simulink model "model4_cm"  (R2018b)
settings: Solver=FixedStepDiscrete  StartTime=0.0  StopTime=Inf  FixedStep=0.025  RelTol=1e-3  EnableMultiTasking=on
undefined symbols (not defined in the file): acA2000, Ace, Basler, FreeRun, ipaddr, PoCL, PTP, USETHISONE
libraries: ptplib x5, dotFinder_ul x2, xpcbitflowlib x1, slrtlib x1, xpcutilitieslib x1, xpcrtudplib x1, videoStream_ul x1, imageUDPNode_ul x1
settings Model: sg_rtwmakecfg_data=_bitflow_  SimulationMode=external  Creator=mcobb  LastModifiedBy=MAE-NCSUCORE
settings SolverCC: ConcurrentTasks=on  AutoInsertRateTranBlk=on
settings DataIOCC: SaveFormat=StructureWithTime
settings OptimizationCC: BlockReduction=off  OptimizeBlockIOStorage=off  BufferReuse=off  GlobalBufferReuse=off  ExpressionFolding=off  LocalBlockOutputs=off  OptimizeDataStoreBuffers=off  BusAssignmentInplaceUpdate=off
settings DebuggingCC: LibraryContextMissingDiagnostic=none
settings HardwareCC: ProdBitPerPointer=32  ProdBitPerSizeT=32  ProdBitPerPtrDiffT=32  ProdLargestAtomicFloat=None  ProdWordSize=32  ProdLongLongMode=on  ProdHWDeviceType=Generic->32-bit x86 compatible
settings SFSimCC: SimUseLocalCustomCode=off
settings RTWCC: SystemTargetFile=slrt.tlc  TemplateMakefile=slrt_default_tmf  Description=Simulink Real-Time  RTWUseLocalCustomCode=off  CodeExecutionProfiling=on  RTWCompilerOptimization=on
settings SimulinkRealTimeCC: SupportVariableSizeSignals=on  PreserveStateflowLocalDataDimensions=off  RL32LogTETModifier=off  xPCisDefaultEnv=off  xPCTargetPCEnvName=Machine4  xPCConcurrentTasks=on

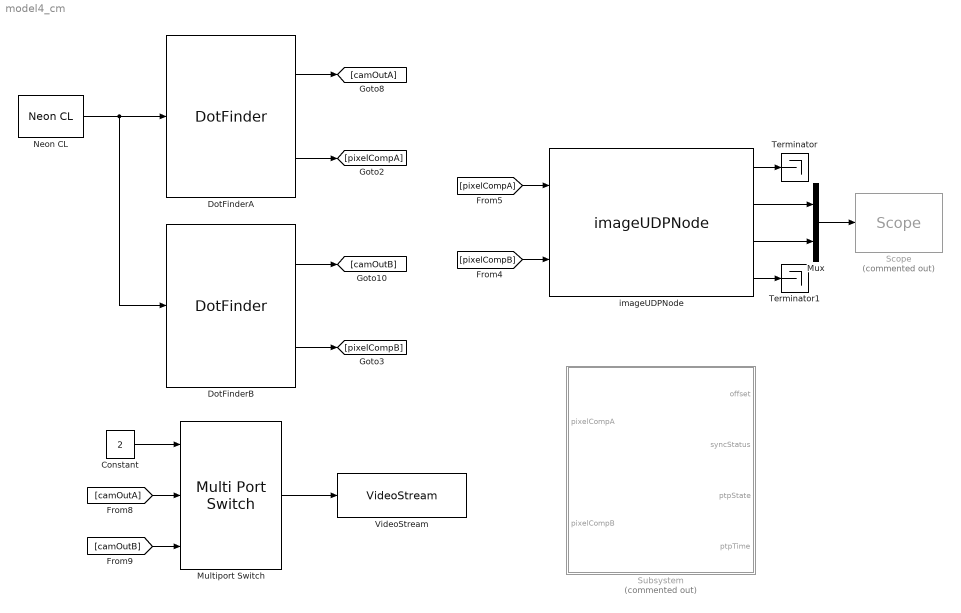
== system model4_cm ==
  Constant : Constant  Value=2
  DotFinderA : dotFinder_ul/DotFinder  ROIPositionHoldEnable=off  InitialCondition=[615 1220]  ROIPositionHoldCoordinates=[615 1220]  ROIDimVec_px=2*[90 30]  ROIHalfDimVec_px=[90 30]  ROISplitDims_px=[1 90 ; 1 60 ; 91 89 ; 1 60]  DotOrientation=Vertical  OverlayOutput=on  ImageDimensions=[1088 2048]  CrosshairPixelWidth_px=1
  DotFinderB : dotFinder_ul/DotFinder  ROIPositionHoldEnable=off  InitialCondition=[465 1200]  ROIPositionHoldCoordinates=[465 1200]  ROIDimVec_px=1.8*[30 90]  ROIHalfDimVec_px=[27 81]  ROISplitDims_px=[1 54 ; 1 81 ; 1 54 ; 82 80]  DotOrientation=Horizontal  OverlayOutput=on  ImageDimensions=[1088 2048]  CrosshairPixelWidth_px=1
  Multiport Switch : MultiPortSwitch  Inputs=2
  Mux : Mux  Inputs=2
  "Neon CL " : xpcbitflowlib/Neon CL   camerapath=Basler-Ace-acA2000-340km-E2-PoCL-FreeRun-USETHISONE.r64  r64=CAMERA  sampletime=0.025  slot=-1  make=Basler  model=acA2000-340km  mode=8 bit, 2 tap, 2048x1088, Free Run  owner=BitFlow  revision=1  modelcomp=0  revcomp=0  aqtimeout=4096  format=1  flashmux=Mux_2TOEP  flashdcc=DCC  pixbitdepth=8  xsize=2048  ysize=1088  xstart=0  ystart=0  dx=2048  dy=1088  expmod="[1  0]"  config="[4294967295         128;4294967295           0;4294967295           0;4294967295           0;4294967295           0;4294967295           0;4294967295      262144;4294967295           0;4294967295           0;4294967295           0;4294967295        1024;4294967295           0;4294967295           0;4294967295  4294967295;4294967295           0;4294967295           0;4294967295           0;4294967295      737280;4294967295        1088;4294967295           0;4294967295           0;4294967295           0;4294967295           0;4294967295           0;4294967295           0;4294967295           0;4294967295        7372;4294967295           0]"  ctab="[4      0     16      1   4112      2     16  32768      0]"  qtabmodel="[1   2048  65536]"  trigmode=0  baud=1  bytewidth=4  parity=1  stopbits=1  command="\"\""  response=0  comments=|
      | Free Run Mode / CC Trigger Mode
      | 
      | CC Trigger can be adjusted via GPV0 in CTAB
      | 
      | To use CC Trigger, camera must set to CC Trigger Mode.
      settings: SourceProductName=Simulink Real-Time: Speedgoat I/O Driver Library
  "Scope " : slrtlib/Displays and Logging/Scope   Commented=on  scopeno=2  scopetype=Target  autostart=on  viewmode=Numerical  formatstr='%15.6f'  grid=on  ylimits=[0,0]  nosamples=250  noprepostsamples=0  interleave=1  triggermode=FreeRun  triggersignal=1  trigsignalfromport=off  triggerlevel=0.0  triggerslope=Either  triggerscope=1  triggersample=0  filename=data.dat  mode=Lazy  writesize=512  autorestart=off  dynamicfilemode=off  maxwritefilesize=512*1024^2
  Subsystem : Subsystem  Commented=on  TreatAsAtomicUnit=on
  Terminator : Terminator
  Terminator1 : Terminator
  VideoStream : videoStream_ul/VideoStream  enbl=on  decimationFactor=5  resizeFactor=1200
  imageUDPNode : imageUDPNode_ul/imageUDPNode  sample_time=0.025  IpAddress=30.30.30.2  toPort=8002  offset_threshold=250e-6  sync_interval=0.2  min_pdelay_req_interval=2.5  MaskUnpackedDataTypes={['double'],['double']}
  wires:
  DotFinderA/2 -> [pixelCompA]
  DotFinderB/2 -> [pixelCompB]
  Constant/1 -> Multiport Switch/1
  Multiport Switch/1 -> VideoStream/1
  [camOutA] -> Multiport Switch/2
  [camOutB] -> Multiport Switch/3
  Mux/1 -> "Scope "/1
  imageUDPNode/3 -> Mux/2
  [pixelCompB] -> imageUDPNode/2
  [pixelCompA] -> imageUDPNode/1
  "Neon CL "/1 -> DotFinderB/1, DotFinderA/1
  DotFinderA/1 -> [camOutA]
  DotFinderB/1 -> [camOutB]
  imageUDPNode/1 -> Terminator/1
  imageUDPNode/4 -> Terminator1/1
  imageUDPNode/2 -> Mux/1

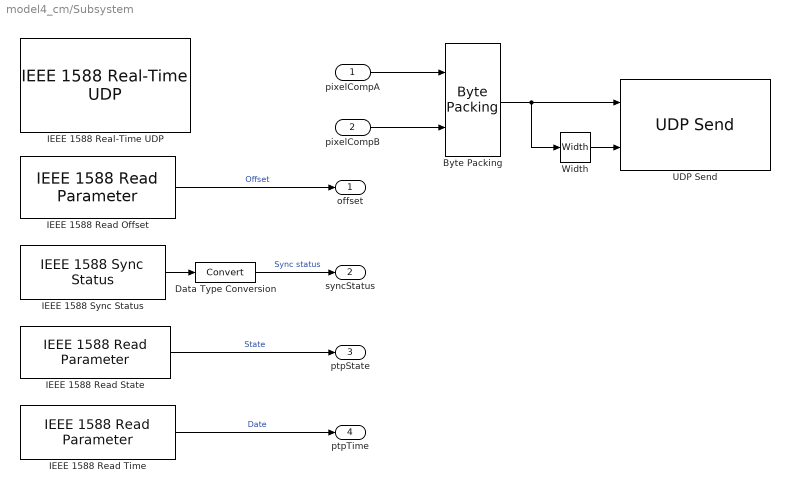
== system model4_cm/Subsystem ==
  pixelCompA : Inport
  pixelCompB : Inport  Port=2
  Byte Packing : xpcutilitieslib/Byte Packing   MaskPackedDataType=uint8  MaskUnpackedDataTypes={['double'],['double']}  MaskAlignment=1
  Data Type Conversion : DataTypeConversion
  IEEE 1588 Read Offset : ptplib/IEEE 1588 Read Parameter  Priority=1  ID=1  param=Offset from Master  sample_time=0.025  enable_read_precision=off
      settings: SourceProductName=Simulink Real-Time  SourceProductBaseCode=XP
  IEEE 1588 Read State : ptplib/IEEE 1588 Read Parameter  Priority=1  ID=1  param=Protocol state  sample_time=0.025  enable_read_precision=off
      settings: SourceProductName=Simulink Real-Time  SourceProductBaseCode=XP
  IEEE 1588 Read Time : ptplib/IEEE 1588 Read Parameter  Priority=1  ID=1  param=PTP time (time-of-day)  sample_time=0.025  enable_read_precision=off
      settings: SourceProductName=Simulink Real-Time  SourceProductBaseCode=XP
  IEEE 1588 Real-Time UDP : ptplib/IEEE 1588 Real-Time UDP  Priority=0  ID=1  PciBus=4  PciSlot=0  PciFunction=0  time_inc=4000000  sample_time=0.025  IpSource=Specify  IpAddress=30.30.30.2  SubnetMask=255.255.255.0  Gateway=0.0.0.0  Receive1=30.30.30.30  dest_ip_select=Standard PTP multicast (224.0.1.129, 224.0.0.107)  custom_dest_ip_addr=30.30.30.30  MulticastList=[ipaddr('224.0.1.129'), ipaddr('224.0.0.107')]  Multicast={macaddr('01:00:5E:00:01:81'), macaddr('01:00:5E:00:00:6B')}  time_source=Ethernet board  timescale=PTP (1970-01-01)  epoch=[1970 01 01 00]  delay_measure=Request-response  slave_only=off  enable_advanced_config=on  domain_num=0  utc_offset=35  priority1=128  clock_class=248  clock_accuracy=hex2dec('FE')  priority2=128  announce_interval=1  sync_interval=0.2  min_pdelay_req_interval=2.5  announce_receipt_timeout=30
      settings: SourceProductName=Simulink Real-Time  SourceProductBaseCode=XP
  IEEE 1588 Sync Status : ptplib/IEEE 1588 Sync Status  Priority=1  ID=1  offset_threshold=250e-6  sample_time=0.025
      settings: SourceProductName=Simulink Real-Time  SourceProductBaseCode=XP
  UDP Send : xpcrtudplib/UDP Send  ipAddressVal=Use host-target connection  localPort=-1  toAddress=30.30.30.30  toPort=8002  sampleTime=0.025
      settings: SourceProductName=Simulink Real-Time  SourceProductBaseCode=XP
  Width : Width
  offset : Outport
  syncStatus : Outport  Port=2
  ptpState : Outport  Port=3
  ptpTime : Outport  Port=4
  wires:
  Data Type Conversion/1 -> syncStatus/1  "Sync status"
  IEEE 1588 Sync Status/1 -> Data Type Conversion/1
  IEEE 1588 Read Time/1 -> ptpTime/1  "Date"
  IEEE 1588 Read State/1 -> ptpState/1  "State"
  IEEE 1588 Read Offset/1 -> offset/1  "Offset"
  Byte Packing/1 -> Width/1, UDP Send/1
  pixelCompB/1 -> Byte Packing/2
  Width/1 -> UDP Send/2
  pixelCompA/1 -> Byte Packing/1
